simulink model "GR_sim"  (R2020a)
settings: Solver=FixedStepAuto  StartTime=0.0  StopTime=10.0  FixedStep=0.01  RelTol=1e-3
InitFcn:
  | GR_Parameters;
values from neighbouring files (symbols this model uses):
  p0 = [1,2]    [GR_Parameters.m]
  R0 = [cos(psi0) -sin(psi0) ... (first row only)    [GR_Parameters.m]
libraries: simulink x1
settings Model: Creator=vcichella  LastModifiedBy=vcichella
settings SFSimCC: CustomCodeUndefinedFunction=UseInterfaceOnly

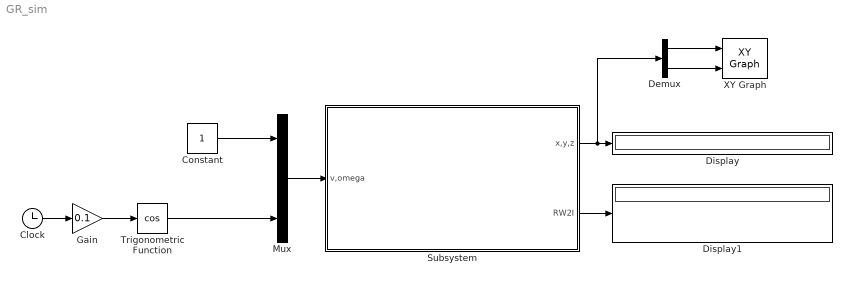
== system GR_sim ==
  Clock : Clock
  Constant : Constant
  Demux : Demux  Outputs=2
  Display : Display
  Display1 : Display
  Gain : Gain  Gain=0.1
  Mux : Mux  Inputs=3
  Subsystem : Subsystem
  Trigonometric Function : Trigonometry  Operator=cos
  XY Graph : simulink/Sinks/XY Graph  xmin=-10  xmax=10  ymin=-10  ymax=10  st=-1
  wires:
  Mux/1 -> Subsystem/1(v,omega)
  Subsystem/1(x,y,z) -> Demux/1, Display/1
  Subsystem/2(RW2I) -> Display1/1
  Constant/1 -> Mux/1
  Trigonometric Function/1 -> Mux/3
  Gain/1 -> Trigonometric Function/1
  Clock/1 -> Gain/1
  Demux/1 -> XY Graph/1
  Demux/2 -> XY Graph/2

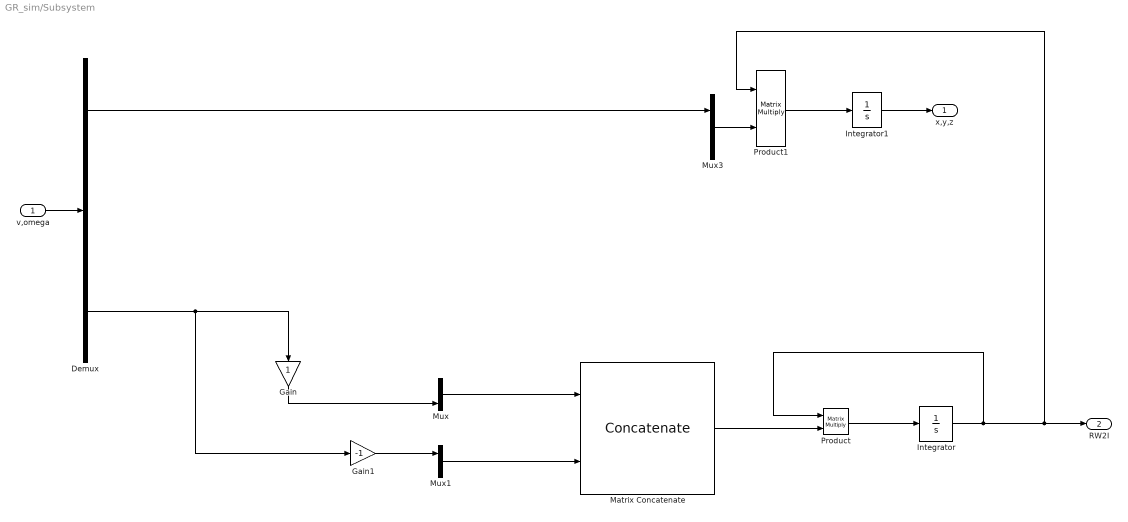
== system GR_sim/Subsystem ==
  v,omega : Inport
  Demux : Demux  Outputs=3
  Gain : Gain
  Gain1 : Gain  Gain=-1
  Integrator : Integrator  InitialCondition=R0
  Integrator1 : Integrator  InitialCondition=p0
  Matrix Concatenate : Concatenate  Mode=Multidimensional array  ConcatenateDimension=2
  Mux : Mux  Inputs=2
  Mux1 : Mux  Inputs=2
  Mux3 : Mux  Inputs=2
  Product : Product  Multiplication=Matrix(*)
  Product1 : Product  Multiplication=Matrix(*)
  x,y,z : Outport  VectorParamsAs1DForOutWhenUnconnected=off
  RW2I : Outport  Port=2  VectorParamsAs1DForOutWhenUnconnected=off
  wires:
  Matrix Concatenate/1 -> Product/2
  v,omega/1 -> Demux/1
  Mux/1 -> Matrix Concatenate/1
  Demux/3 -> Gain1/1, Gain/1
  Product/1 -> Integrator/1
  Demux/1 -> Mux3/1
  Integrator1/1 -> x,y,z/1
  Product1/1 -> Integrator1/1
  Integrator/1 -> Product1/1, RW2I/1, Product/1
  Mux3/1 -> Product1/2
  Gain/1 -> Mux/2
  Gain1/1 -> Mux1/1
  Mux1/1 -> Matrix Concatenate/2
